simulink model "Mod4VidAincomplete"  (R2022b)
settings: Solver=FixedStepAuto  StartTime=0.0  StopTime=inf  RelTol=1e-3  EnableMultiTasking=on
libraries: vexarmcortexlib x17, vexcommonlib x1, RoboticsPlayground x1
settings Model: Creator=carol  LastModifiedBy=carol
settings DataIOCC: LimitDataPoints=on  SignalLoggingSaveFormat=ModelDataLogs  ReturnWorkspaceOutputs=off
settings OptimizationCC: ExpressionDepthLimit=2147483647  LifeSpan=Inf  MaxStackSize=64  EfficientTunableParamExpr=on
settings DebuggingCC: UnderspecifiedInitializationDetection=Classic  MergeDetectMultiDrivingBlocksExec=none  InheritedTsInSrcMsg=none  FcnCallInpInsideContextMsg=warning  StateNameClashWarn=warning  SFUnexpectedBacktrackingDiag=warning  SFNoUnconditionalDefaultTransitionDiag=warning  SFExecutionAtInitializationDiag=none  SFMachineParentedDataDiag=warning  ArithmeticOperatorsInVariantConditions=warning
settings HardwareCC: ProdBitPerPointer=32  ProdBitPerSizeT=32  ProdBitPerPtrDiffT=32  ProdLargestAtomicInteger=Long  ProdLargestAtomicFloat=Double  ProdIntDivRoundTo=Undefined  ProdWordSize=32  ProdHWDeviceType=ARM Compatible->ARM Cortex
settings ModelReferenceCC: EnableRefExpFcnMdlSchedulingChecks=on  PropagateSignalLabelsOutOfModel=off
settings SFSimCC: MATLABDynamicMemAlloc=off  CustomCodeUndefinedFunction=UseInterfaceOnly
settings RTWCC: Description=Embedded Coder  SystemTargetFile=ert.tlc  HardwareBoard=ARM Cortex-based VEX Microcontroller  TemplateMakefile=ert_default_tmf  Toolchain=GNU Tools for VEX ARM Cortex
settings CodeAppCC: IgnoreCustomStorageClasses=off  CustomSymbolStrType=$N$R$M  StateflowObjectComments=on  InternalIdentifier=Classic
settings ERTTargetCC: CodeReplacementLibrary=GCC ARM Cortex-M3  MultiwordLength=2048  ConvertIfToSwitch=off  SuppressUnreachableDefaultCases=off

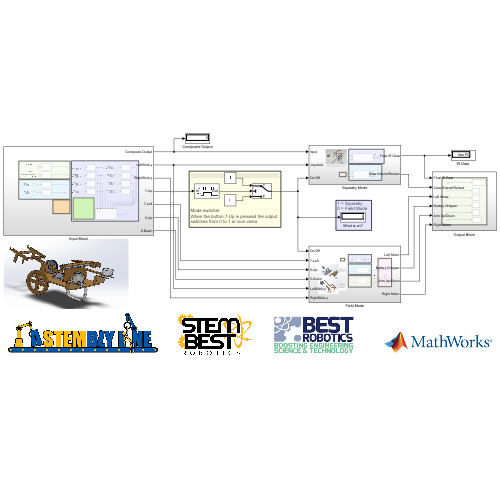
[thumbnail: Simulink's stored preview of the top-level diagram]
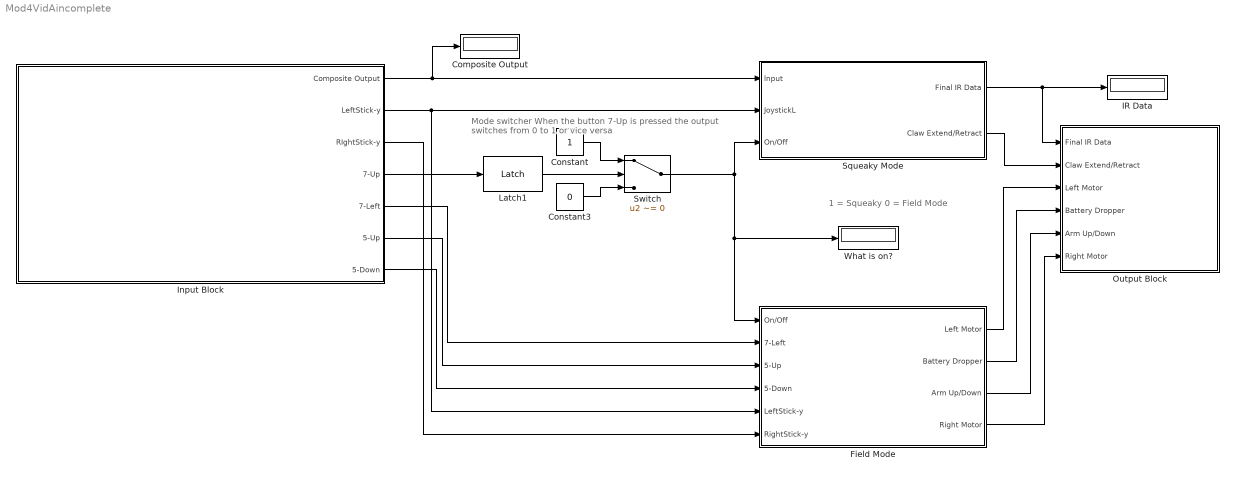
== system Mod4VidAincomplete ==
  note: 1 = Squeaky
      | 0 = Field Mode
  note: Mode switcher
      | When the button 7-Up is pressed the output
      | switches from 0 to 1 or vice versa
  Composite Output : Display
  Constant : Constant
  Constant3 : Constant  Value=0
  Field Mode : Subsystem
  "IR Data " : Display
      settings: Format=hex (Stored Integer)
  Input Block : Subsystem
  Latch1 : RoboticsPlayground/Utilities and Hardware/Latch  SystemSampleTime=-1  VariantActivationTime=update diagram  Latency=0  AutoFrameSizeCalculation=off
      settings: SourceProductName=Robotics Playground
  Output Block : Subsystem
  Squeaky Mode : Subsystem
  Switch : Switch  Criteria=u2 ~= 0  SaturateOnIntegerOverflow=off  InputSameDT=off
  What is on? : Display
  wires:
  Switch/1 -> Squeaky Mode/3(On/Off), Field Mode/1(On/Off), What is on?/1
  Constant3/1 -> Switch/3
  Latch1/1 -> Switch/2
  Input Block/1(Composite Output) -> Squeaky Mode/1(lnput), Composite Output/1
  Input Block/4(7-Up) -> Latch1/1
  Constant/1 -> Switch/1
  Input Block/2(LeftStick-y) -> Squeaky Mode/2(JoystickL), Field Mode/5(LeftStick-y)
  Field Mode/1(Left Motor) -> Output Block/3(Left Motor)
  Field Mode/2(Battery Dropper) -> Output Block/4(Battery Dropper)
  Field Mode/4(Right Motor) -> Output Block/6(Right Motor)
  Field Mode/3(Arm Up/Down) -> Output Block/5("Arm Up/Down ")
  Input Block/3(RIghtStick-y) -> Field Mode/6(RightStick-y)
  Input Block/7(5-Down) -> Field Mode/4(5-Down)
  Input Block/6(5-Up) -> Field Mode/3(5-Up)
  Input Block/5(7-Left) -> Field Mode/2(7-Left)
  Squeaky Mode/1(Final IR Data) -> "IR Data "/1, Output Block/1(Final IR Data)
  Squeaky Mode/2(Claw Extend/Retract) -> Output Block/2(Claw Extend/Retract)

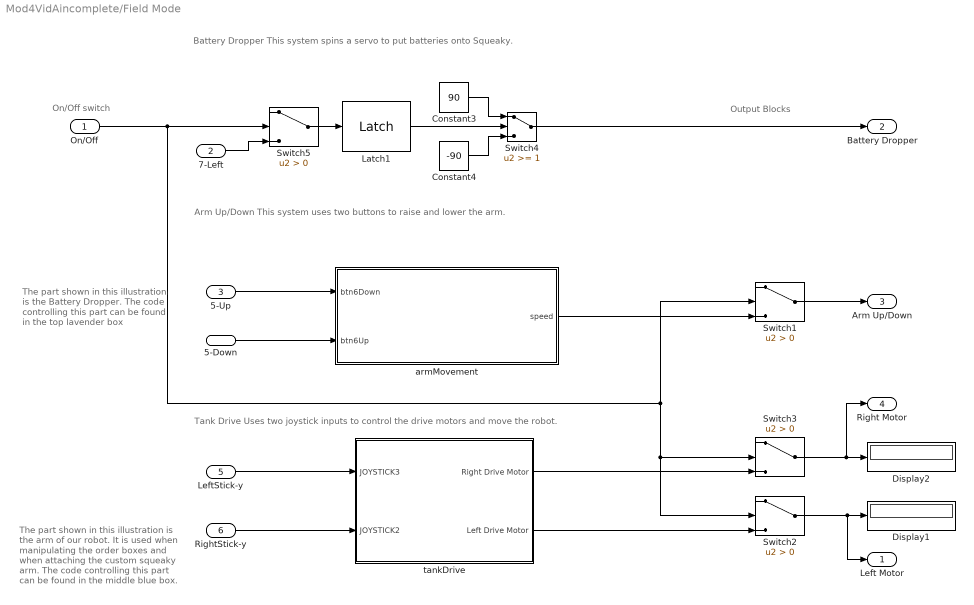
== system Mod4VidAincomplete/Field Mode ==
  note: The part shown in this illustration is the arm of our robot. It is used when
      | manipulating the order boxes and when attaching the custom squeaky arm. The code controlling this part can be found in the middle blue box.
  note: The part shown in this illustration is the Battery Dropper. The code controlling this part can be found in the top lavender box
  note: Output Blocks
  note: Battery Dropper
      | This system spins a servo to put batteries onto Squeaky.
  note: Tank Drive
      | Uses two joystick inputs to control the drive motors and move the robot.
  note: Arm Up/Down
      | This system uses two buttons to raise and lower the arm.
  note: On/Off switch
  On/Off : Inport
  7-Left : Inport  Port=2
  5-Up : Inport  Port=3
  5-Down : Inport  Port=4
  LeftStick-y : Inport  Port=5
  RightStick-y : Inport  Port=6
  Constant3 : Constant  Value=90
  Constant4 : Constant  Value=-90
  Display1 : Display
  Display2 : Display
  Latch1 : vexcommonlib/Latch  output0=off  BlockPlatform=vexarmcortex
  Switch{1..3,5} (4 alike) : Switch  Criteria=u2 > Threshold  SaturateOnIntegerOverflow=off  InputSameDT=off
  Switch4 : Switch  Threshold=1  SaturateOnIntegerOverflow=off  InputSameDT=off
  armMovement : Stateflow chart  TreatAsAtomicUnit=on
  "tankDrive " : Subsystem  TreatAsAtomicUnit=on
  Left Motor : Outport
  Battery Dropper : Outport  Port=2
  Arm Up/Down : Outport  Port=3
  Right Motor : Outport  Port=4
  wires:
  5-Down/1 -> armMovement/2(btn6Up)
  5-Up/1 -> armMovement/1(btn6Down)
  Latch1/1 -> Switch4/2
  Constant4/1 -> Switch4/3
  RightStick-y/1 -> "tankDrive "/2(JOYSTICK2)
  "tankDrive "/1(Right Drive Motor) -> Switch3/3
  LeftStick-y/1 -> "tankDrive "/1(JOYSTICK3)
  armMovement/1(speed) -> Switch1/3
  Constant3/1 -> Switch4/1
  "tankDrive "/2(Left Drive Motor) -> Switch2/3
  On/Off/1 -> Switch2/2, Switch3/2, Switch1/2, Switch5/2
  Switch1/1 -> Arm Up/Down/1
  Switch3/1 -> Right Motor/1, Display2/1
  Switch2/1 -> Left Motor/1, Display1/1
  Switch4/1 -> Battery Dropper/1
  Switch5/1 -> Latch1/1
  7-Left/1 -> Switch5/3

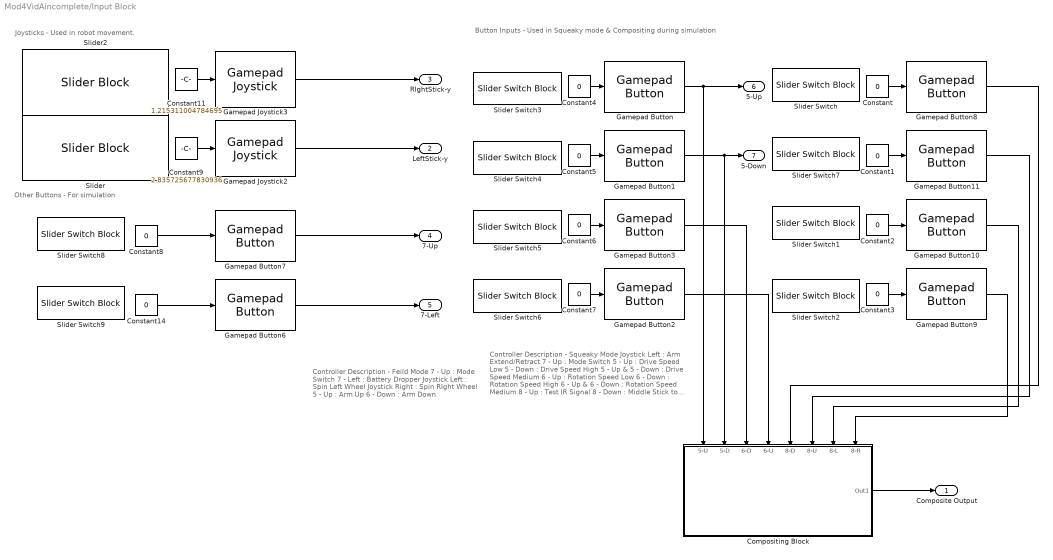
== system Mod4VidAincomplete/Input Block ==
  note: Controller Description - Feild Mode
      |
      | 7 - Up : Mode Switch
      | 7 - Left : Battery Dropper
      |
      | Joystick Left : Spin Left Wheel
      | Joystick Right : Spin RIght Wheel
      |
      | 5 - Up : Arm Up
      | 6 - Down : Arm Down
  note: Controller  Description - Squeaky Mode
      |
      | Joystick Left : Arm Extend/Retract
      |
      |  7 - Up : Mode Switch
      |
      | 5 - Up : Drive Speed Low
      | 5 - Down : Drive Speed High
      | 5 - Up & 5 - Down : Drive Speed Medium
      |
      | 6 - Up : Rotation Speed Low
      | 6 - Down : Rotation Speed High
      | 6 - Up & 6 - Down : Rotation Speed Medium
      |
      | 8 - Up : Test IR Signal
      | 8 - Down : Middle Stick to Drive
      | 8 - Right : Middle Stick to Rotate
      | 8 - Left : Middle Stick to Lift
  note: Other Buttons - For simulation
  note: Button Inputs - Used in Squeaky mode & Compositing during simulation
  note: Joysticks - Used in robot movement.
  Compositing Block : Subsystem
      settings: PortSchema="{\"entries\":[{\"content\":{\"sides\":[{\"content\":{\"connectorIds\":[]},\"type\":\"ConnectorPlacement.EquallySpacedRectSide\",\"uuid\":\"9d2b5337-c4d4-4923-a699-a47fc21a7185\"},{\"content\":{\"connectorIds\":[\"Out1\"],\"side\":\"RIGHT\"},\"type\":\"ConnectorPlacement.EquallySpacedRectSide\",\"uuid\":\"56c06069-3940-4c56-b8fd-a4c3d4ffc63d\"},{\"content\":{\"connectorIds\":[\"In1\",\"In2\",\"In3\",\"In4\",\"In5\",\"In6\",\"In7\",\"In8\"],\"side\":\"TOP\"},\"type\":\"ConnectorPlacement.EquallySpacedRectSide\",\"uuid\":\"14368183-39e9-4405-bfbf-e8557249760c\"}]},\"type\":\"ConnectorPlacement.EquallySpacedConnector\",\"uuid\":\"5d0b0675-df6a-4749-851b-50901843da5f\"}],\"packageUris\":[\"http://schema.mathworks.com/mf0/Connector/R2020b\"],\"version\":\"1.0\"}"
  Constant{,1..8,14} (10 alike) : Constant  Value=0
  Constant11 : Constant  Value=1.215311004784695
  Constant9 : Constant  Value=2.835725677830936
  Gamepad Button : vexarmcortexlib/Gamepad/Gamepad Button  joystick=1  chan=5  button56=Up  button78=Down  SimulationIn=on  SampleTime=0.02
  Gamepad Button1 : vexarmcortexlib/Gamepad/Gamepad Button  joystick=1  chan=5  button56=Down  button78=Down  SimulationIn=on  SampleTime=0.02
  Gamepad Button10 : vexarmcortexlib/Gamepad/Gamepad Button  joystick=1  chan=8  button56=Up  button78=Left  SimulationIn=on  SampleTime=0.02
  Gamepad Button11 : vexarmcortexlib/Gamepad/Gamepad Button  joystick=1  chan=8  button56=Up  button78=Up  SimulationIn=on  SampleTime=0.02
  Gamepad Button2 : vexarmcortexlib/Gamepad/Gamepad Button  joystick=1  chan=6  button56=Up  button78=Down  SimulationIn=on  SampleTime=0.02
  Gamepad Button3 : vexarmcortexlib/Gamepad/Gamepad Button  joystick=1  chan=6  button56=Down  button78=Down  SimulationIn=on  SampleTime=0.02
  Gamepad Button6 : vexarmcortexlib/Gamepad/Gamepad Button  joystick=1  chan=7  button56=Up  button78=Left  SimulationIn=on  SampleTime=0.02
  Gamepad Button7 : vexarmcortexlib/Gamepad/Gamepad Button  joystick=1  chan=7  button56=Up  button78=Up  SimulationIn=on  SampleTime=0.02
  Gamepad Button8 : vexarmcortexlib/Gamepad/Gamepad Button  joystick=1  chan=8  button56=Up  button78=Down  SimulationIn=on  SampleTime=0.02
  Gamepad Button9 : vexarmcortexlib/Gamepad/Gamepad Button  joystick=1  chan=8  button56=Up  button78=Right  SimulationIn=on  SampleTime=0.02
  Gamepad Joystick2 : vexarmcortexlib/Gamepad/Gamepad Joystick  joystick=1  chan=3  SimulationIn=on  SampleTime=0.02
  Gamepad Joystick3 : vexarmcortexlib/Gamepad/Gamepad Joystick  joystick=1  chan=2  SimulationIn=on  SampleTime=0.02
  Slider : SliderBlock  ScaleMin=-127  ScaleMax=127
  Slider Switch{,1..9} (10 alike) : SliderSwitchBlock
      settings: Values={{'Off', 'On'}, [0 1]}
  Slider2 : SliderBlock  ScaleMin=-127  ScaleMax=127
  Composite Output : Outport
  LeftStick-y : Outport  Port=2
  RIghtStick-y : Outport  Port=3
  7-Up : Outport  Port=4
  7-Left : Outport  Port=5
  5-Up : Outport  Port=6
  5-Down : Outport  Port=7
  wires:
  Gamepad Button7/1 -> 7-Up/1
  Gamepad Button6/1 -> 7-Left/1
  Constant/1 -> Gamepad Button8/1
  Constant1/1 -> Gamepad Button11/1
  Constant2/1 -> Gamepad Button10/1
  Constant3/1 -> Gamepad Button9/1
  Constant4/1 -> Gamepad Button/1
  Constant5/1 -> Gamepad Button1/1
  Constant7/1 -> Gamepad Button2/1
  Constant6/1 -> Gamepad Button3/1
  Constant8/1 -> Gamepad Button7/1
  Compositing Block/1(Out1) -> Composite Output/1
  Constant9/1 -> Gamepad Joystick2/1
  Gamepad Button/1 -> 5-Up/1, Compositing Block/1(5-U)
  Gamepad Button1/1 -> 5-Down/1, Compositing Block/2(5-D)
  Gamepad Button3/1 -> Compositing Block/3(6-D)
  Gamepad Button2/1 -> Compositing Block/4(6-U)
  Gamepad Button8/1 -> Compositing Block/5(8-D)
  Gamepad Button11/1 -> Compositing Block/6(8-U)
  Gamepad Button10/1 -> Compositing Block/7(8-L)
  Gamepad Button9/1 -> Compositing Block/8(8-R)
  Constant11/1 -> Gamepad Joystick3/1
  Gamepad Joystick3/1 -> RIghtStick-y/1
  Gamepad Joystick2/1 -> LeftStick-y/1
  Constant14/1 -> Gamepad Button6/1

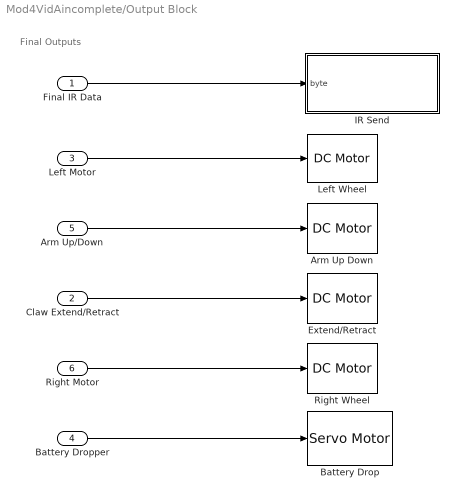
== system Mod4VidAincomplete/Output Block ==
  note: Final Outputs
  Final IR Data : Inport
  Claw Extend/Retract : Inport  Port=2
  Left Motor : Inport  Port=3
  Battery Dropper : Inport  Port=4
  "Arm Up/Down " : Inport  Port=5
  Right Motor : Inport  Port=6
  Arm Up Down : vexarmcortexlib/Actuators/DC Motor  motor=4  scaleFactor=1/13.5  SimulationOut=off
  Battery Drop : vexarmcortexlib/Actuators/Servo Motor  motor=3  scaleFactor=60/127  SimulationOut=off
  Extend/Retract : vexarmcortexlib/Actuators/DC Motor  motor=6  scaleFactor=1/13.5  SimulationOut=off
  IR Send : Subsystem
  Left Wheel : vexarmcortexlib/Actuators/DC Motor  motor=2  scaleFactor=1/13.5  SimulationOut=off
  Right Wheel : vexarmcortexlib/Actuators/DC Motor  motor=9  scaleFactor=1/13.5  SimulationOut=off
  wires:
  Final IR Data/1 -> IR Send/1(byte)
  Claw Extend/Retract/1 -> Extend/Retract/1
  Left Motor/1 -> Left Wheel/1
  Battery Dropper/1 -> Battery Drop/1
  Right Motor/1 -> Right Wheel/1
  "Arm Up/Down "/1 -> Arm Up Down/1

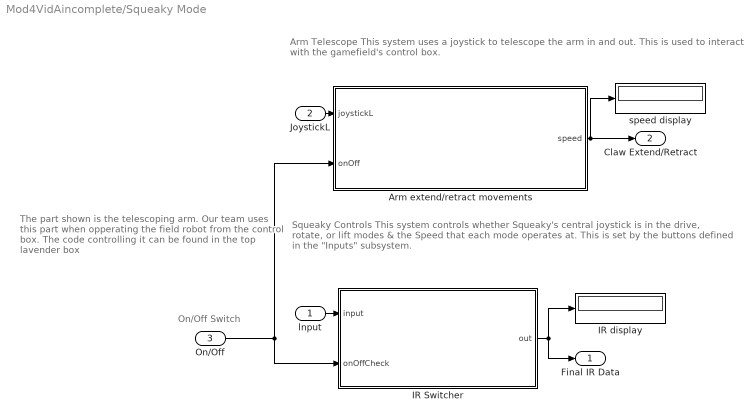
== system Mod4VidAincomplete/Squeaky Mode ==
  note: The part shown is the telescoping arm. Our team uses this
      | part when opperating the field robot from the control box.
      | The code controlling it can be found in the top lavender box
  note: On/Off Switch
  note: Squeaky Controls
      | This system controls whether Squeaky's central joystick is in the drive,
      |  rotate, or lift modes & the Speed that each mode operates at. This is set
      |  by the buttons defined in the "Inputs" subsystem.
  note: Arm Telescope
      | This system uses a joystick to telescope the arm in and out.
      | This is used to interact with the gamefield's control box.
  lnput : Inport
  JoystickL : Inport  Port=2
  On/Off : Inport  Port=3
  Arm extend/retract movements : Stateflow chart  TreatAsAtomicUnit=on
  IR Switcher : Stateflow chart  TreatAsAtomicUnit=on
  IR display : Display
      settings: Format=hex (Stored Integer)
  speed display : Display
  Final IR Data : Outport
  Claw Extend/Retract : Outport  Port=2
  wires:
  On/Off/1 -> IR Switcher/2(onOffCheck), Arm extend/retract movements/2(onOff)
  lnput/1 -> IR Switcher/1(input)
  JoystickL/1 -> Arm extend/retract movements/1(joystickL)
  Arm extend/retract movements/1(speed) -> Claw Extend/Retract/1, speed display/1
  IR Switcher/1(out) -> IR display/1, Final IR Data/1

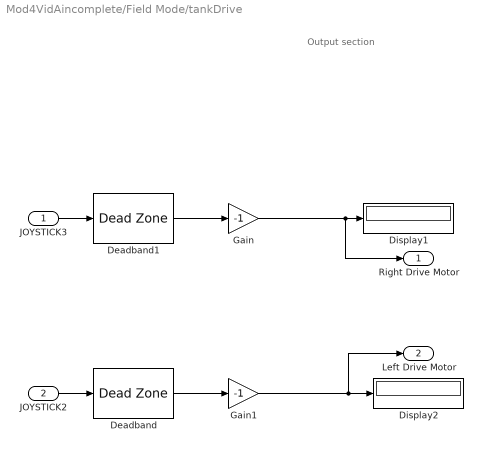
== system Mod4VidAincomplete/Field Mode/tankDrive  ==
  note: Output section
  JOYSTICK3 : Inport
  JOYSTICK2 : Inport  Port=2
  Deadband : DeadZone  LowerValue=-9  UpperValue=9
  Deadband1 : DeadZone  LowerValue=-9  UpperValue=9
  Display1 : Display
  Display2 : Display
  Gain : Gain  Gain=-1
  Gain1 : Gain  Gain=-1
  Right Drive Motor : Outport
  Left Drive Motor : Outport  Port=2
  wires:
  JOYSTICK3/1 -> Deadband1/1
  Gain/1 -> Right Drive Motor/1, Display1/1
  Gain1/1 -> Display2/1, Left Drive Motor/1
  JOYSTICK2/1 -> Deadband/1
  Deadband1/1 -> Gain/1
  Deadband/1 -> Gain1/1

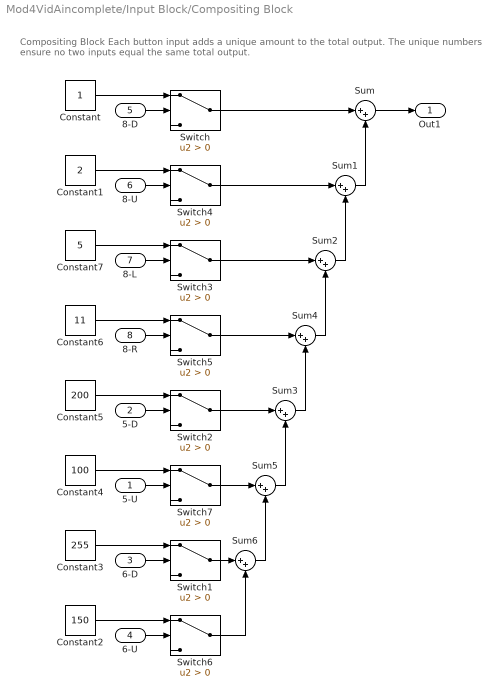
== system Mod4VidAincomplete/Input Block/Compositing Block ==
  note: Compositing Block
      | Each button input adds a unique amount to the total output. The unique numbers
      | ensure no two inputs equal the same total output.
  5-U : Inport
  5-D : Inport  Port=2
  6-D : Inport  Port=3
  6-U : Inport  Port=4
  8-D : Inport  Port=5
  8-U : Inport  Port=6
  8-L : Inport  Port=7
  8-R : Inport  Port=8
  Constant : Constant
  Constant1 : Constant  Value=2
  Constant2 : Constant  Value=150
  Constant3 : Constant  Value=255
  Constant4 : Constant  Value=100
  Constant5 : Constant  Value=200
  Constant6 : Constant  Value=11
  Constant7 : Constant  Value=5
  Sum{,1..6} (7 alike) : Sum  Inputs=|++
  Switch{,1..7} (8 alike) : Switch  Criteria=u2 > Threshold  SaturateOnIntegerOverflow=off  InputSameDT=off
  Out1 : Outport
  wires:
  8-D/1 -> Switch/2
  Sum/1 -> Out1/1
  Switch4/1 -> Sum1/1
  Sum1/1 -> Sum/2
  Switch3/1 -> Sum2/1
  Sum2/1 -> Sum1/2
  Switch5/1 -> Sum4/1
  Switch6/1 -> Sum6/2
  Switch1/1 -> Sum6/1
  Switch7/1 -> Sum5/1
  Switch2/1 -> Sum3/1
  Sum4/1 -> Sum2/2
  Sum3/1 -> Sum4/2
  Sum5/1 -> Sum3/2
  Sum6/1 -> Sum5/2
  Switch/1 -> Sum/1
  8-U/1 -> Switch4/2
  8-L/1 -> Switch3/2
  6-U/1 -> Switch6/2
  6-D/1 -> Switch1/2
  5-U/1 -> Switch7/2
  5-D/1 -> Switch2/2
  8-R/1 -> Switch5/2
  Constant/1 -> Switch/1
  Constant1/1 -> Switch4/1
  Constant7/1 -> Switch3/1
  Constant5/1 -> Switch2/1
  Constant6/1 -> Switch5/1
  Constant2/1 -> Switch6/1
  Constant4/1 -> Switch7/1
  Constant3/1 -> Switch1/1

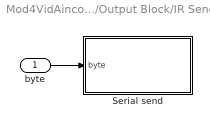
== system Mod4VidAincomplete/Output Block/IR Send ==
  byte : Inport  OutDataTypeStr=uint8  PortDimensions=[1 1]
  Serial send : MATLAB Function  TreatAsAtomicUnit=on
  wires:
  byte/1 -> Serial send/1(byte)

== stateflow chart Mod4VidAincomplete/Field Mode/armMovement ==
  state ARMDOWN
    entry:
    speed = -50;
  state STOPPED
    entry:
    speed = 0;
  state ARMUP
    entry:
    speed = 140;
  (default) -> STOPPED
  STOPPED -> ARMUP [order 1] : [btn6Down == 0 && btn6Up == 1 ]
  STOPPED -> ARMDOWN [order 2] : [btn6Down == 1 && btn6Up == 0]
  ARMDOWN -> STOPPED [order 2] : [btn6Down == 0]
  ARMUP -> STOPPED [order 2] : [btn6Up == 0]
  ARMDOWN -> STOPPED [order 1] : [btn6Down == 1 && btn6Up == 1]
  ARMUP -> STOPPED [order 1] : [btn6Down == 1 && btn6Up == 1]
  data: speed output; btn6Down input; btn6Up input

== stateflow chart Mod4VidAincomplete/Squeaky Mode/Arm extend//retract movements ==
  state armExtend
    entry:
    speed = 80;
  state noArm
    entry:
    speed = 0;
  state armRetract
    entry:
    speed = -80;
  (default) -> noArm
  noArm -> armRetract [order 1] : [joystickL <= -10 && onOff == 1]
  noArm -> armExtend [order 2] : [joystickL >= 10 && onOff == 1]
  armRetract -> noArm : [joystickL >= 10 | onOff == 0]
  armExtend -> noArm : [joystickL <= 10 | onOff ==0]
  data: speed output; joystickL input; onOff input

== matlab function Mod4VidAincomplete/Output Block/IR Send/Serial send ==
  data: byte input
function fcn(byte)
% Serial send single byte
%#codegen

% Config
port = 'uart1';
baud = uint32(600);

persistent isFirstRun

if coder.target('Rtw')
    coder.cinclude('API.h');
    coder.cinclude('string.h');
    file = coder.opaque('FILE *', port,'HeaderFile','API.h');

    if isempty(isFirstRun)
        % first time setup
        isFirstRun = false;

        flags = coder.opaque('uint16', 'SERIAL_8N1');
        coder.ceval('usartInit', file, baud, flags);
    end

    coder.ceval('fputc', byte, file);

end

end

== stateflow chart Mod4VidAincomplete/Squeaky Mode/IR Switcher ==
  state Drive Speed Adjustments [group]
    state drivespeedHigh
      entry:
      out = 0xC3;
    state drivespeedLow
      entry:
      out = 0x99;
    state drivespeedMed
      entry:
      out = 0xA5;
  state onOff
    entry:
    out = 0x00;
  state Squeaky Movements [group]
    state lift_2
      entry:
      out = 0x5A;
    state drive_2
      entry:
      out = 0x3C;
    state rotate_2
      entry:
      out = 0x33;
  state irTestDefault
    entry:
    out = 0xF0;
  state Rotational Adjustments [group]
    state rotatespeedHigh
      entry:
      out = 0x0F;
    state rotatespeedLow
      entry:
      out = 0x69;
    state rotatespeedMed
      entry:
      out = 0x96;
  (default) -> onOff
  irTestDefault -> drivespeedHigh [order 5] : [input == 100]
  drivespeedHigh -> irTestDefault : [input ~= 100 | onOffCheck == 0]
  onOff -> irTestDefault : [onOffCheck == 1]
  irTestDefault -> onOff [order 2] : [onOffCheck == 0]
  irTestDefault -> drivespeedLow [order 8] : [input == 200]
  irTestDefault -> lift_2 [order 1] : [input == 5]
  drivespeedLow -> irTestDefault : [input ~= 200|onOffCheck == 0]
  lift_2 -> irTestDefault : [input ~= 5|onOffCheck == 0]
  irTestDefault -> drivespeedMed [order 9] : [input==300]
  drivespeedMed -> irTestDefault : [input ~= 300|onOffCheck == 0]
  rotatespeedHigh -> irTestDefault : [input ~= 150|onOffCheck == 0]
  irTestDefault -> drive_2 [order 3] : [input == 1]
  drive_2 -> irTestDefault : [input ~=1|onOffCheck == 0]
  irTestDefault -> rotatespeedHigh [order 7] : [input == 150]
  irTestDefault -> rotatespeedLow [order 6] : [input == 255]
  rotatespeedLow -> irTestDefault : [input ~= 250|onOffCheck == 0]
  irTestDefault -> rotatespeedMed [order 10] : [input == 405]
  rotatespeedMed -> irTestDefault : [input ~= 405|onOffCheck == 0]
  rotate_2 -> irTestDefault : [input ~= 11|onOffCheck == 0]
  irTestDefault -> rotate_2 [order 4] : [input == 11]
  data: input input; out output; onOffCheck input
